simulink model "npc_controller"  (R2022a)
settings: Solver=FixedStepDiscrete  StartTime=0.0  StopTime=20  RelTol=1e-3  EnableMultiTasking=on
values from neighbouring files (symbols this model uses):
  Tsw = 1.5E-5    [param.sldd]
undefined symbols (not defined in the file or in its folder): CAN_O_INT, CANA_BASE, Down, GPTRIP1SEL, GPTRIP2SEL, GPTRIP3SEL, TZ1, TZ2, TZ3, Up
libraries: simulink x153, hdlsllib x90, c2802xlib x34, c2837xDlib x18, c280xlib x12, canmsglib x9, c2838xlib x8, idelinklib_common x3, c2806xlib x2, slpidlib x2, c28004xlib x2, c281xlib x2
(part 32 of 45)

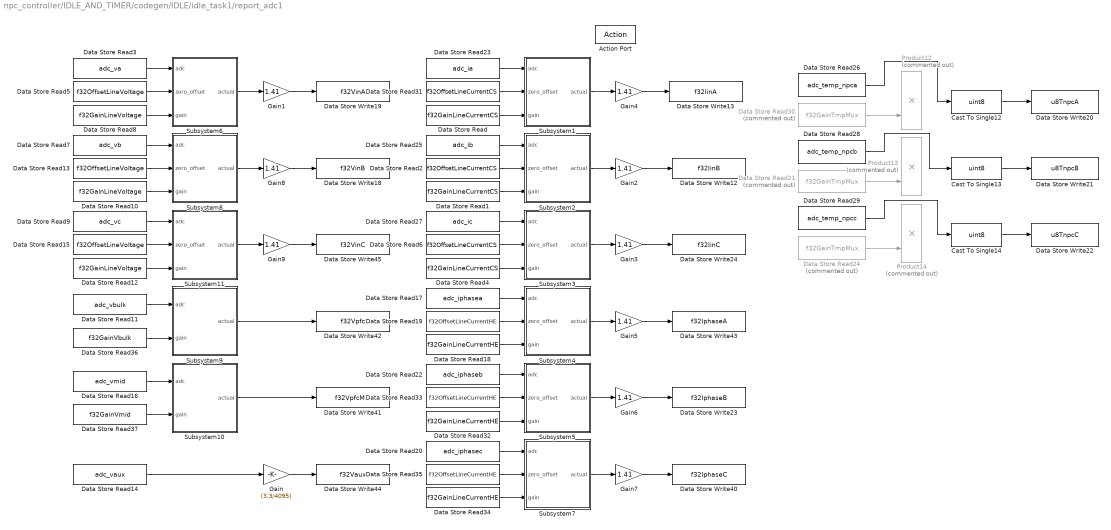
== system npc_controller/IDLE_AND_TIMER/codegen/IDLE/idle_task1/report_adc1 ==
  Action Port : ActionPort
  Cast To Single12 : DataTypeConversion  OutDataTypeStr=uint8  SaturateOnIntegerOverflow=off  RndMeth=Floor
  Cast To Single13 : DataTypeConversion  OutDataTypeStr=uint8  SaturateOnIntegerOverflow=off  RndMeth=Floor
  Cast To Single14 : DataTypeConversion  OutDataTypeStr=uint8  SaturateOnIntegerOverflow=off  RndMeth=Floor
  Data Store Read : DataStoreRead  DataStoreName=f32GainLineCurrentCS  IndexOptions=Index vector (dialog)  Indices=1  OutputSizes=1
  Data Store Read1 : DataStoreRead  DataStoreName=f32GainLineCurrentCS  IndexOptions=Index vector (dialog)  Indices=1  OutputSizes=1
  Data Store Read10 : DataStoreRead  DataStoreName=f32GainLineVoltage  IndexOptions=Index vector (dialog)  Indices=1  OutputSizes=1
  Data Store Read11 : DataStoreRead  DataStoreName=adc_vbulk  IndexOptions=Index vector (dialog)  Indices=1  OutputSizes=1
  Data Store Read12 : DataStoreRead  DataStoreName=f32GainLineVoltage  IndexOptions=Index vector (dialog)  Indices=1  OutputSizes=1
  Data Store Read13 : DataStoreRead  DataStoreName=f32OffsetLineVoltage  IndexOptions=Index vector (dialog)  Indices=1  OutputSizes=1
  Data Store Read14 : DataStoreRead  DataStoreName=adc_vaux  IndexOptions=Index vector (dialog)  Indices=1  OutputSizes=1
  Data Store Read15 : DataStoreRead  DataStoreName=f32OffsetLineVoltage  IndexOptions=Index vector (dialog)  Indices=1  OutputSizes=1
  Data Store Read16 : DataStoreRead  DataStoreName=adc_vmid  IndexOptions=Index vector (dialog)  Indices=1  OutputSizes=1
  Data Store Read17 : DataStoreRead  DataStoreName=adc_iphasea  IndexOptions=Index vector (dialog)  Indices=1  OutputSizes=1
  Data Store Read18 : DataStoreRead  DataStoreName=f32GainLineCurrentHE  IndexOptions=Index vector (dialog)  Indices=1  OutputSizes=1
  Data Store Read19 : DataStoreRead  DataStoreName=f32OffsetLineCurrentHE  IndexOptions=Index vector (dialog)  Indices=1  OutputSizes=1
  Data Store Read2 : DataStoreRead  DataStoreName=f32OffsetLineCurrentCS  IndexOptions=Index vector (dialog)  Indices=1  OutputSizes=1
  Data Store Read20 : DataStoreRead  DataStoreName=adc_iphasec  IndexOptions=Index vector (dialog)  Indices=1  OutputSizes=1
  Data Store Read21 : DataStoreRead  Commented=on  DataStoreName=f32GainTmpMux  IndexOptions=Index vector (dialog)  Indices=1  OutputSizes=1
  Data Store Read22 : DataStoreRead  DataStoreName=adc_iphaseb  IndexOptions=Index vector (dialog)  Indices=1  OutputSizes=1
  Data Store Read23 : DataStoreRead  DataStoreName=adc_ia  IndexOptions=Index vector (dialog)  Indices=1  OutputSizes=1
  Data Store Read24 : DataStoreRead  Commented=on  DataStoreName=f32GainTmpMux  IndexOptions=Index vector (dialog)  Indices=1  OutputSizes=1
  Data Store Read25 : DataStoreRead  DataStoreName=adc_ib  IndexOptions=Index vector (dialog)  Indices=1  OutputSizes=1
  Data Store Read26 : DataStoreRead  DataStoreName=adc_temp_npca  IndexOptions=Index vector (dialog)  Indices=1  OutputSizes=1
  Data Store Read27 : DataStoreRead  DataStoreName=adc_ic  IndexOptions=Index vector (dialog)  Indices=1  OutputSizes=1
  Data Store Read28 : DataStoreRead  DataStoreName=adc_temp_npcb  IndexOptions=Index vector (dialog)  Indices=1  OutputSizes=1
  Data Store Read29 : DataStoreRead  DataStoreName=adc_temp_npcc  IndexOptions=Index vector (dialog)  Indices=1  OutputSizes=1
  Data Store Read3 : DataStoreRead  DataStoreName=adc_va  IndexOptions=Index vector (dialog)  Indices=1  OutputSizes=1
  Data Store Read30 : DataStoreRead  Commented=on  DataStoreName=f32GainTmpMux  IndexOptions=Index vector (dialog)  Indices=1  OutputSizes=1
  Data Store Read31 : DataStoreRead  DataStoreName=f32OffsetLineCurrentCS  IndexOptions=Index vector (dialog)  Indices=1  OutputSizes=1
  Data Store Read32 : DataStoreRead  DataStoreName=f32GainLineCurrentHE  IndexOptions=Index vector (dialog)  Indices=1  OutputSizes=1
  Data Store Read33 : DataStoreRead  DataStoreName=f32OffsetLineCurrentHE  IndexOptions=Index vector (dialog)  Indices=1  OutputSizes=1
  Data Store Read34 : DataStoreRead  DataStoreName=f32GainLineCurrentHE  IndexOptions=Index vector (dialog)  Indices=1  OutputSizes=1
  Data Store Read35 : DataStoreRead  DataStoreName=f32OffsetLineCurrentHE  IndexOptions=Index vector (dialog)  Indices=1  OutputSizes=1
  Data Store Read36 : DataStoreRead  DataStoreName=f32GainVbulk  IndexOptions=Index vector (dialog)  Indices=1  OutputSizes=1
  Data Store Read37 : DataStoreRead  DataStoreName=f32GainVmid  IndexOptions=Index vector (dialog)  Indices=1  OutputSizes=1
  Data Store Read4 : DataStoreRead  DataStoreName=f32GainLineCurrentCS  IndexOptions=Index vector (dialog)  Indices=1  OutputSizes=1
  Data Store Read5 : DataStoreRead  DataStoreName=f32OffsetLineVoltage  IndexOptions=Index vector (dialog)  Indices=1  OutputSizes=1
  Data Store Read6 : DataStoreRead  DataStoreName=f32OffsetLineCurrentCS  IndexOptions=Index vector (dialog)  Indices=1  OutputSizes=1
  Data Store Read7 : DataStoreRead  DataStoreName=adc_vb  IndexOptions=Index vector (dialog)  Indices=1  OutputSizes=1
  Data Store Read8 : DataStoreRead  DataStoreName=f32GainLineVoltage  IndexOptions=Index vector (dialog)  Indices=1  OutputSizes=1
  Data Store Read9 : DataStoreRead  DataStoreName=adc_vc  IndexOptions=Index vector (dialog)  Indices=1  OutputSizes=1
  Data Store Write12 : DataStoreWrite  DataStoreName=f32IinB  IndexOptions=Index vector (dialog)  Indices=1  OutputSizes=1
  Data Store Write13 : DataStoreWrite  DataStoreName=f32IinA  IndexOptions=Index vector (dialog)  Indices=1  OutputSizes=1
  Data Store Write18 : DataStoreWrite  DataStoreName=f32VinB  IndexOptions=Index vector (dialog)  Indices=1  OutputSizes=1
  Data Store Write19 : DataStoreWrite  DataStoreName=f32VinA  IndexOptions=Index vector (dialog)  Indices=1  OutputSizes=1
  Data Store Write20 : DataStoreWrite  DataStoreName=u8TnpcA  IndexOptions=Index vector (dialog)  Indices=1  OutputSizes=1
  Data Store Write21 : DataStoreWrite  DataStoreName=u8TnpcB  IndexOptions=Index vector (dialog)  Indices=1  OutputSizes=1
  Data Store Write22 : DataStoreWrite  DataStoreName=u8TnpcC  IndexOptions=Index vector (dialog)  Indices=1  OutputSizes=1
  Data Store Write23 : DataStoreWrite  DataStoreName=f32IphaseB  IndexOptions=Index vector (dialog)  Indices=1  OutputSizes=1
  Data Store Write24 : DataStoreWrite  DataStoreName=f32IinC  IndexOptions=Index vector (dialog)  Indices=1  OutputSizes=1
  Data Store Write40 : DataStoreWrite  DataStoreName=f32IphaseC  IndexOptions=Index vector (dialog)  Indices=1  OutputSizes=1
  Data Store Write41 : DataStoreWrite  DataStoreName=f32VpfcMid  IndexOptions=Index vector (dialog)  Indices=1  OutputSizes=1
  Data Store Write42 : DataStoreWrite  DataStoreName=f32Vpfc  IndexOptions=Index vector (dialog)  Indices=1  OutputSizes=1
  Data Store Write43 : DataStoreWrite  DataStoreName=f32IphaseA  IndexOptions=Index vector (dialog)  Indices=1  OutputSizes=1
  Data Store Write44 : DataStoreWrite  DataStoreName=f32Vaux  IndexOptions=Index vector (dialog)  Indices=1  OutputSizes=1
  Data Store Write45 : DataStoreWrite  DataStoreName=f32VinC  IndexOptions=Index vector (dialog)  Indices=1  OutputSizes=1
  Gain : Gain  Gain=(3.3/4095)  ParamDataTypeStr=single  OutDataTypeStr=single
  Gain{1..9} (9 alike) : Gain  Gain=1.41  ParamDataTypeStr=single  OutDataTypeStr=single
  Product12 : Product  Commented=on  OutDataTypeStr=single
  Product13 : Product  Commented=on  OutDataTypeStr=single
  Product14 : Product  Commented=on  OutDataTypeStr=single
  Subsystem1 : Subsystem
  Subsystem10 : Subsystem
  Subsystem11 : Subsystem
  Subsystem2 : Subsystem
  Subsystem3 : Subsystem
  Subsystem4 : Subsystem
  Subsystem5 : Subsystem
  Subsystem6 : Subsystem
  Subsystem7 : Subsystem
  Subsystem8 : Subsystem
  Subsystem9 : Subsystem
  wires:
  Data Store Read3/1 -> Subsystem6/1(adc)
  Subsystem8/1(actual) -> Gain8/1
  Subsystem11/1(actual) -> Gain9/1
  Subsystem5/1(actual) -> Gain6/1
  Subsystem7/1(actual) -> Gain7/1
  Subsystem4/1(actual) -> Gain5/1
  Subsystem3/1(actual) -> Gain3/1
  Subsystem2/1(actual) -> Gain2/1
  Gain7/1 -> Data Store Write40/1
  Gain6/1 -> Data Store Write23/1
  Gain5/1 -> Data Store Write43/1
  Gain3/1 -> Data Store Write24/1
  Subsystem9/1(actual) -> Data Store Write42/1
  Data Store Read23/1 -> Subsystem1/1(adc)
  Gain1/1 -> Data Store Write19/1
  Subsystem6/1(actual) -> Gain1/1
  Gain2/1 -> Data Store Write12/1
  Gain4/1 -> Data Store Write13/1
  Subsystem10/1(actual) -> Data Store Write41/1
  Gain9/1 -> Data Store Write45/1
  Gain8/1 -> Data Store Write18/1
  Data Store Read29/1 -> Cast To Single14/1
  Data Store Read28/1 -> Cast To Single13/1
  Data Store Read26/1 -> Cast To Single12/1
  Data Store Read13/1 -> Subsystem8/2(zero_offset)
  Data Store Read10/1 -> Subsystem8/3(gain)
  Data Store Read31/1 -> Subsystem1/2(zero_offset)
  Data Store Read/1 -> Subsystem1/3(gain)
  Data Store Read8/1 -> Subsystem6/3(gain)
  Data Store Read5/1 -> Subsystem6/2(zero_offset)
  Gain/1 -> Data Store Write44/1
  Data Store Read37/1 -> Subsystem10/2(gain)
  Data Store Read36/1 -> Subsystem9/2(gain)
  Data Store Read12/1 -> Subsystem11/3(gain)
  Data Store Read15/1 -> Subsystem11/2(zero_offset)
  Data Store Read16/1 -> Subsystem10/1(adc)
  Data Store Read11/1 -> Subsystem9/1(adc)
  Data Store Read9/1 -> Subsystem11/1(adc)
  Data Store Read7/1 -> Subsystem8/1(adc)
  Data Store Read34/1 -> Subsystem7/3(gain)
  Data Store Read35/1 -> Subsystem7/2(zero_offset)
  Data Store Read33/1 -> Subsystem5/2(zero_offset)
  Data Store Read32/1 -> Subsystem5/3(gain)
  Data Store Read18/1 -> Subsystem4/3(gain)
  Data Store Read19/1 -> Subsystem4/2(zero_offset)
  Data Store Read4/1 -> Subsystem3/3(gain)
  Data Store Read6/1 -> Subsystem3/2(zero_offset)
  Data Store Read1/1 -> Subsystem2/3(gain)
  Data Store Read2/1 -> Subsystem2/2(zero_offset)
  Data Store Read20/1 -> Subsystem7/1(adc)
  Data Store Read22/1 -> Subsystem5/1(adc)
  Data Store Read17/1 -> Subsystem4/1(adc)
  Data Store Read27/1 -> Subsystem3/1(adc)
  Data Store Read25/1 -> Subsystem2/1(adc)
  Subsystem1/1(actual) -> Gain4/1
  Data Store Read24/1 -> Product14/2
  Data Store Read21/1 -> Product13/2
  Data Store Read30/1 -> Product12/2
  Cast To Single12/1 -> Data Store Write20/1
  Cast To Single14/1 -> Data Store Write22/1
  Cast To Single13/1 -> Data Store Write21/1
  Data Store Read14/1 -> Gain/1

== system npc_controller/IDLE_AND_TIMER/codegen/IDLE/idle_task1/set_tmp_mux ==
  Action Port : ActionPort  ActionPortLabel=case [ 3 ]:
  Function-Call Generator : simulink/Ports & Subsystems/Function-Call Generator  sample_time=-1  numberOfIterations=1  DisallowWideOutput=off
  Function-Call Split : FunctionCallSplit  NumOutputPorts=2
  Function-Call Split1 : FunctionCallSplit  NumOutputPorts=2
  incr_cnt_tmp_mux : Subsystem  TreatAsAtomicUnit=on
      settings: RTWSystemCode=Inline
  parse_cnt_tmp_mux : Subsystem  TreatAsAtomicUnit=on
      settings: RTWSystemCode=Inline
  set_tmp_mux : Subsystem
  wires:
  Function-Call Generator/1 -> Function-Call Split/1
  Function-Call Split/1 -> parse_cnt_tmp_mux/Trigger
  Function-Call Split1/2 -> incr_cnt_tmp_mux/Trigger
  Function-Call Split1/1 -> set_tmp_mux/Trigger
  Function-Call Split/2 -> Function-Call Split1/1

== system npc_controller/IDLE_AND_TIMER/codegen/IDLE/idle_task1/watchdog ==
  note: Note add MLE
  Action Port : ActionPort  ActionPortLabel=case [ 0 ]:
  Watchdog : c281xlib/Watchdog  resetsrc=Specify via dialog  sample=-1
      settings: SourceProductBaseCode=TIC2000

== system npc_controller/IDLE_AND_TIMER/codegen/INITIALIZATION/clb/System Initialize1 ==

== system npc_controller/IDLE_AND_TIMER/codegen/INITIALIZATION/clb/System Initialize2 ==

== system npc_controller/IDLE_AND_TIMER/codegen/INITIALIZATION/clb/System Initialize8 ==

== system npc_controller/IDLE_AND_TIMER/codegen/INITIALIZATION/epwm/System Initialize3 ==

== system npc_controller/IDLE_AND_TIMER/codegen/INITIALIZATION/epwm1/System Initialize1 ==

== system npc_controller/IDLE_AND_TIMER/codegen/INITIALIZATION/epwm1/System Initialize3 ==

== system npc_controller/IDLE_AND_TIMER/codegen/INITIALIZATION/outputxbar/System Initialize1 ==

== system npc_controller/IDLE_AND_TIMER/codegen/INITIALIZATION/outputxbar/System Initialize2 ==

== system npc_controller/IDLE_AND_TIMER/codegen/INITIALIZATION/outputxbar/System Initialize3 ==

== system npc_controller/IDLE_AND_TIMER/codegen/INITIALIZATION/outputxbar/System Initialize4 ==

== system npc_controller/IDLE_AND_TIMER/codegen/INITIALIZATION/outputxbar/System Initialize5 ==

== system npc_controller/IDLE_AND_TIMER/codegen/INITIALIZATION/outputxbar/System Initialize6 ==

== system npc_controller/IDLE_AND_TIMER/codegen/INITIALIZATION/outputxbar/System Initialize7 ==

== system npc_controller/IDLE_AND_TIMER/codegen/TIMER_100MS/incr_cnt/inc ==
  Action Port : ActionPort  ActionPortLabel=else
  Add : Sum
  Constant : Constant  OutDataTypeStr=uint16
  Data Store Read : DataStoreRead  DataStoreName=cnt_poll_can_msg  IndexOptions=Index vector (dialog)  Indices=1  OutputSizes=1
  Data Store Write : DataStoreWrite  DataStoreName=cnt_poll_can_msg  IndexOptions=Index vector (dialog)  Indices=1  OutputSizes=1
  wires:
  Add/1 -> Data Store Write/1
  Data Store Read/1 -> Add/1
  Constant/1 -> Add/2

== system npc_controller/IDLE_AND_TIMER/codegen/TIMER_100MS/incr_cnt/reset ==
  Action Port : ActionPort  ActionPortLabel=if(u1 > 10)
  Constant : Constant  Value=0  OutDataTypeStr=uint16
  Data Store Write : DataStoreWrite  DataStoreName=cnt_poll_can_msg  IndexOptions=Index vector (dialog)  Indices=1  OutputSizes=1
  wires:
  Constant/1 -> Data Store Write/1

== system npc_controller/IDLE_AND_TIMER/codegen/TIMER_1MS/codegen/periodic_timer1 ==
  note: Note:
      |  - Worst error of tfv is timer interval (1ms) + twice the execution of supervisory loop
      |  - Effective max count is 65.536 = 2e16*1e-3
  Add : Sum  Commented=on
  Add1 : Sum
  Constant : Constant  Commented=on  OutDataTypeStr=uint16
  Constant1 : Constant  OutDataTypeStr=uint16
  Data Store Read : DataStoreRead  Commented=on  DataStoreName=cnt_1ms  IndexOptions=Index vector (dialog)  Indices=1  OutputSizes=1
  Data Store Read1 : DataStoreRead  DataStoreName=cnt_1ms  IndexOptions=Index vector (dialog)  Indices=1  OutputSizes=1
  Data Store Write : DataStoreWrite  Commented=on  DataStoreName=cnt_1ms  IndexOptions=Index vector (dialog)  Indices=1  OutputSizes=1
  Data Store Write1 : DataStoreWrite  DataStoreName=cnt_1ms  IndexOptions=Index vector (dialog)  Indices=1  OutputSizes=1
  Rate Transition2 : RateTransition
  Rate Transition3 : RateTransition
  wires:
  Constant/1 -> Add/2
  Add/1 -> Data Store Write/1
  Data Store Read/1 -> Add/1
  Rate Transition3/1 -> Add1/1
  Rate Transition2/1 -> Data Store Write1/1
  Data Store Read1/1 -> Rate Transition3/1
  Add1/1 -> Rate Transition2/1
  Constant1/1 -> Add1/2

== system npc_controller/CONTROL/CONTROL/false/CLA_CONTROL/CONTROL/IIR Filter1 ==
  note: prev 0.98
  x[n] : Inport
  1 - Lambda : Gain  Gain=1-0.9996  ParamDataTypeStr=single  OutDataTypeStr=single
  Delay : Delay  DelayLength=1  StateName=vmid_delay2  StateMustResolveToSignalObject=on
  Delay1 : Delay  DelayLength=1  StateName=vmid_delay1  StateMustResolveToSignalObject=on
  Lambda : Gain  Gain=0.9996  ParamDataTypeStr=single  OutDataTypeStr=single
  Sum : Sum  Inputs=|++  AccumDataTypeStr=single  OutDataTypeStr=single
  y[n] : Outport
  wires:
  Delay/1 -> Lambda/1
  Lambda/1 -> Sum/2
  Sum/1 -> y[n]/1, Delay/1
  1 - Lambda/1 -> Sum/1
  x[n]/1 -> Delay1/1
  Delay1/1 -> 1 - Lambda/1

== system npc_controller/CONTROL/CONTROL/false/CLA_CONTROL/CONTROL/IIR Filter3 ==
  note: prev 0.98
  x[n] : Inport
  1 - Lambda : Gain  Gain=1-0.9996  ParamDataTypeStr=single  OutDataTypeStr=single
  Delay : Delay  DelayLength=1  StateName=vbulk_delay2  StateMustResolveToSignalObject=on
  Delay1 : Delay  DelayLength=1  StateName=vbulk_delay1  StateMustResolveToSignalObject=on
  Lambda : Gain  Gain=0.9996  ParamDataTypeStr=single  OutDataTypeStr=single
  Sum : Sum  Inputs=|++  AccumDataTypeStr=single  OutDataTypeStr=single
  y[n] : Outport
  wires:
  Delay/1 -> Lambda/1
  Lambda/1 -> Sum/2
  Sum/1 -> y[n]/1, Delay/1
  1 - Lambda/1 -> Sum/1
  x[n]/1 -> Delay1/1
  Delay1/1 -> 1 - Lambda/1

== system npc_controller/CONTROL/CONTROL/false/CLA_CONTROL/CONTROL/If Action Subsystem ==
  In1 : Inport
  Action Port : ActionPort  ActionPortLabel=if(u1 == 1)
  Out1 : Outport
  wires:
  In1/1 -> Out1/1

== system npc_controller/CONTROL/CONTROL/false/CLA_CONTROL/CONTROL/If Action Subsystem1 ==
  In1 : Inport
  Action Port : ActionPort  ActionPortLabel=else
  Out1 : Outport
  wires:
  In1/1 -> Out1/1

== system npc_controller/CONTROL/CONTROL/false/CLA_CONTROL/CONTROL/Subsystem1 ==
  note: Note:
      | pol_pha
      | 0 - pos
      | 1 - neg
  iLref : Inport
  vbal_coef : Inport  Port=2
  pol : Inport  Port=3
  AND4 : Logic  Operator=NAND  IconShape=distinctive  AllPortsSameDT=off  OutDataTypeStr=boolean
  AND5 : Logic  IconShape=distinctive  AllPortsSameDT=off  OutDataTypeStr=boolean
  Add : Sum  AccumDataTypeStr=single  OutDataTypeStr=single
  Constant4 : Constant  Value=2  OutDataTypeStr=single  SampleTime=-1
  From3 : From  Commented=on  GotoTag=iLref
  From4 : From  Commented=on  GotoTag=iLref_pos
  From5 : From  Commented=on  GotoTag=iLref_neg
  From52 : From  Commented=on  GotoTag=vbal_coef_top
  From53 : From  Commented=on  GotoTag=vbal_coef_bot
  Mux : Mux  Commented=on  Inputs=3
  Mux1 : Mux  Commented=on  Inputs=2
  Product{4..5,10..11} (4 alike) : Product  OutDataTypeStr=single
  Scope3 : Scope  Commented=on  NumInputPorts=2
  delVdc5 : Sum  Inputs=|+-  AccumDataTypeStr=single  OutDataTypeStr=single
  iLref_vbal : Outport
  wires:
  Mux/1 -> Scope3/2
  Mux1/1 -> Scope3/1
  From52/1 -> Mux1/1
  From53/1 -> Mux1/2
  From5/1 -> Mux/3
  From4/1 -> Mux/2
  From3/1 -> Mux/1
  pol/1 -> [pol]
  Add/1 -> iLref_vbal/1
  iLref/1 -> [iLref]
  vbal_coef/1 -> [vbal_coef_top]
  [vbal_coef_top] -> delVdc5/2
  Constant4/1 -> delVdc5/1
  delVdc5/1 -> [vbal_coef_bot]
  [iLref] -> AND5/1, Product11/1
  Product5/1 -> Add/2
  [iLref_pos] -> Product4/1
  [vbal_coef_top] -> Product4/2
  [iLref_neg] -> Product5/1
  AND4/1 -> Product10/2
  Product4/1 -> Add/1
  Product10/1 -> [iLref_pos]
  [pol] -> AND4/2
  [vbal_coef_bot] -> Product5/2
  [iLref] -> AND4/1, Product10/1
  AND5/1 -> Product11/2
  [pol] -> AND5/2
  Product11/1 -> [iLref_neg]

== system npc_controller/CONTROL/CONTROL/false/CLA_CONTROL/CONTROL/Subsystem2 ==
  note: Note:
      | pol_pha
      | 0 - pos
      | 1 - neg
  iLref : Inport
  vbal_coef : Inport  Port=2
  pol : Inport  Port=3
  AND4 : Logic  Operator=NAND  IconShape=distinctive  AllPortsSameDT=off  OutDataTypeStr=boolean
  AND5 : Logic  IconShape=distinctive  AllPortsSameDT=off  OutDataTypeStr=boolean
  Add : Sum  AccumDataTypeStr=single  OutDataTypeStr=single
  Constant4 : Constant  Value=2  OutDataTypeStr=single  SampleTime=-1
  From3 : From  Commented=on  GotoTag=iLref
  From4 : From  Commented=on  GotoTag=iLref_pos
  From5 : From  Commented=on  GotoTag=iLref_neg
  From52 : From  Commented=on  GotoTag=vbal_coef_top
  From53 : From  Commented=on  GotoTag=vbal_coef_bot
  Mux : Mux  Commented=on  Inputs=3
  Mux1 : Mux  Commented=on  Inputs=2
  Product{4..5,10..11} (4 alike) : Product  OutDataTypeStr=single
  Scope3 : Scope  Commented=on  NumInputPorts=2
  delVdc5 : Sum  Inputs=|+-  AccumDataTypeStr=single  OutDataTypeStr=single
  iLref_vbal : Outport
  wires:
  Product11/1 -> [iLref_neg]
  [pol] -> AND5/2
  AND5/1 -> Product11/2
  [iLref] -> Product10/1, AND4/1
  [vbal_coef_bot] -> Product5/2
  [pol] -> AND4/2
  Product10/1 -> [iLref_pos]
  Product4/1 -> Add/1
  AND4/1 -> Product10/2
  [iLref_neg] -> Product5/1
  [vbal_coef_top] -> Product4/2
  [iLref_pos] -> Product4/1
  Product5/1 -> Add/2
  [iLref] -> Product11/1, AND5/1
  delVdc5/1 -> [vbal_coef_bot]
  Constant4/1 -> delVdc5/1
  [vbal_coef_top] -> delVdc5/2
  vbal_coef/1 -> [vbal_coef_top]
  iLref/1 -> [iLref]
  Add/1 -> iLref_vbal/1
  pol/1 -> [pol]
  From3/1 -> Mux/1
  From4/1 -> Mux/2
  From5/1 -> Mux/3
  From53/1 -> Mux1/2
  From52/1 -> Mux1/1
  Mux1/1 -> Scope3/1
  Mux/1 -> Scope3/2

== system npc_controller/CONTROL/CONTROL/false/CLA_CONTROL/CONTROL/Subsystem5 ==
  vxn : Inport  OutDataTypeStr=single
  vbulk : Inport  Port=2  OutDataTypeStr=single
  iLxref : Inport  Port=3  OutDataTypeStr=single
  Constant4 : Constant  OutDataTypeStr=single  SampleTime=-1
  Delay : Delay  DelayLength=1  StateName=dcmccm_delay  StateMustResolveToSignalObject=on
  Divide6 : Product  Inputs=*/  OutDataTypeStr=single
  Divide7 : Product  Inputs=***/  OutDataTypeStr=single
  Gain10 : Gain  Gain=0.5  ParamDataTypeStr=single  OutDataTypeStr=single
  Gain11 : Gain  Gain=1538  ParamDataTypeStr=single  OutDataTypeStr=single
  Gain9 : Gain  Gain=0.0036102/0.001798  ParamDataTypeStr=single  OutDataTypeStr=single
  KL : Constant  Value=2.6305  OutDataTypeStr=single  SampleTime=-1
  Min : MinMax  Inputs=2  OutDataTypeStr=single
  Saturation2 : Saturate  UpperLimit=1  LowerLimit=0  OutDataTypeStr=single
  Saturation3 : Saturate  UpperLimit=1  LowerLimit=0  OutDataTypeStr=single
  Sqrt : Sqrt  OutputSignalType=real  OutDataTypeStr=single  IntermediateResultsDataTypeStr=single
  Sum7 : Sum  Inputs=|+-  AccumDataTypeStr=single  OutDataTypeStr=single
  D_FF : Outport  OutDataTypeStr=single
  wires:
  Gain10/1 -> Divide6/2
  Saturation2/1 -> Delay/1, Min/1  "D_CCM"
  vxn/1 -> Divide7/4, Gain9/1
  Gain9/1 -> Divide6/1
  Sqrt/1 -> Saturation3/1
  Sum7/1 -> Saturation2/1
  Gain11/1 -> D_FF/1  "D_FF"
  Divide7/1 -> Sqrt/1
  Saturation3/1 -> Min/2  "D_DCM"
  Divide6/1 -> Sum7/2
  Constant4/1 -> Sum7/1
  iLxref/1 -> Divide7/3
  Delay/1 -> Divide7/1
  Min/1 -> Gain11/1
  KL/1 -> Divide7/2
  vbulk/1 -> Gain10/1

== system npc_controller/CONTROL/CONTROL/false/CLA_CONTROL/CONTROL/midpoint voltage balancing ==
  note: Note:
      | pol_pha
      | 0 - pos
      | 1 - neg
  iLref : Inport
  vbal_coef : Inport  Port=2
  pol : Inport  Port=3
  AND4 : Logic  Operator=NAND  IconShape=distinctive  AllPortsSameDT=off  OutDataTypeStr=boolean
  AND5 : Logic  IconShape=distinctive  AllPortsSameDT=off  OutDataTypeStr=boolean
  Add : Sum  AccumDataTypeStr=single  OutDataTypeStr=single
  Constant4 : Constant  Value=2  OutDataTypeStr=single  SampleTime=-1
  From3 : From  Commented=on  GotoTag=iLref
  From4 : From  Commented=on  GotoTag=iLref_pos
  From5 : From  Commented=on  GotoTag=iLref_neg
  From52 : From  Commented=on  GotoTag=vbal_coef_top
  From53 : From  Commented=on  GotoTag=vbal_coef_bot
  Mux : Mux  Commented=on  Inputs=3
  Mux1 : Mux  Commented=on  Inputs=2
  Product{4..5,10..11} (4 alike) : Product  OutDataTypeStr=single
  Scope3 : Scope  Commented=on  NumInputPorts=2
  delVdc5 : Sum  Inputs=|+-  AccumDataTypeStr=single  OutDataTypeStr=single
  iLref_vbal : Outport
  wires:
  Product11/1 -> [iLref_neg]
  [pol] -> AND5/2
  AND5/1 -> Product11/2
  [iLref] -> Product10/1, AND4/1
  [vbal_coef_bot] -> Product5/2
  [pol] -> AND4/2
  Product10/1 -> [iLref_pos]
  Product4/1 -> Add/1
  AND4/1 -> Product10/2
  [iLref_neg] -> Product5/1
  [vbal_coef_top] -> Product4/2
  [iLref_pos] -> Product4/1
  Product5/1 -> Add/2
  [iLref] -> Product11/1, AND5/1
  delVdc5/1 -> [vbal_coef_bot]
  Constant4/1 -> delVdc5/1
  [vbal_coef_top] -> delVdc5/2
  vbal_coef/1 -> [vbal_coef_top]
  iLref/1 -> [iLref]
  Add/1 -> iLref_vbal/1
  pol/1 -> [pol]
  From3/1 -> Mux/1
  From4/1 -> Mux/2
  From5/1 -> Mux/3
  From53/1 -> Mux1/2
  From52/1 -> Mux1/1
  Mux1/1 -> Scope3/1
  Mux/1 -> Scope3/2

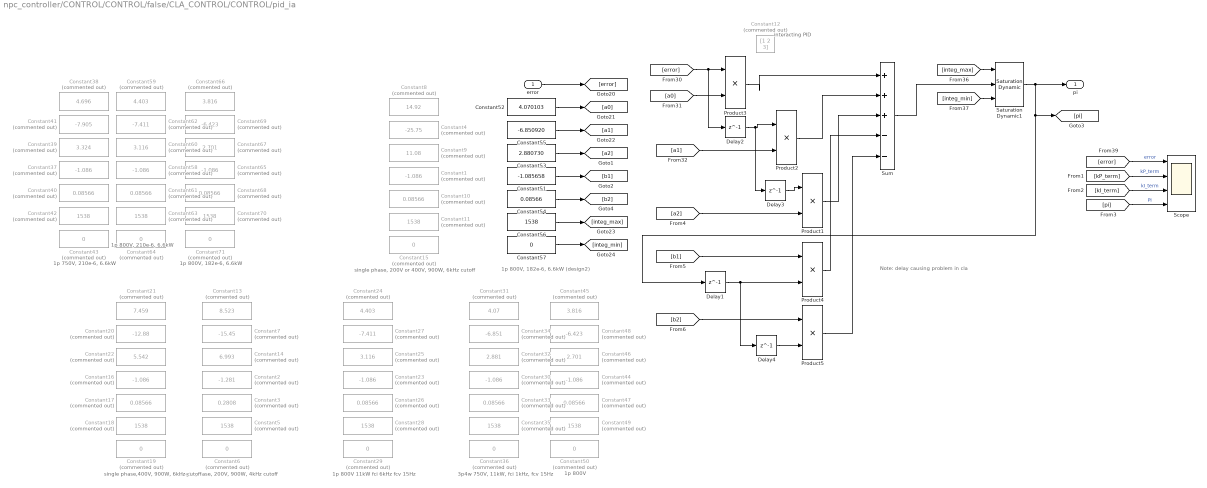
== system npc_controller/CONTROL/CONTROL/false/CLA_CONTROL/CONTROL/pid_ia ==
  note: single phase, 200V or 400V, 900W, 6kHz cutoff
  note: interacting PID
  note: Note: delay causing problem in cla
  note: single phase, 200V, 900W, 4kHz cutoff
  note: single phase,400V, 900W, 6kHz cutoff
  note: 1p 800V 11kW fci 6kHz fcv 15Hz
  note: 3p4w 750V, 11kW, fci 1kHz, fcv 15Hz
  note: 1p 750V, 210e-6, 6.6kW
  note: 1p 800V
  note: 1p 800V, 182e-6, 6.6kW (design2)
  note: 1p 800V, 210e-6, 6.6kW
  note: 1p 800V, 182e-6, 6.6kW
  error : Inport  OutDataTypeStr=single
  Constant{1,16,23,30,37,44,58,65} (8 alike) : Constant  Commented=on  Value=-1.086  OutDataTypeStr=single
  Constant{10,17,26,33,40,47,61,68} (8 alike) : Constant  Commented=on  Value=0.08566  OutDataTypeStr=single
  Constant{5,11,18,28,35,42,49,63,70} (9 alike) : Constant  Commented=on  Value=1538  OutDataTypeStr=single
  Constant12 : Constant  Commented=on  Value=[1 2 3]  OutDataTypeStr=single
  Constant13 : Constant  Commented=on  Value=8.523  VectorParams1D=off  OutDataTypeStr=single
  Constant14 : Constant  Commented=on  Value=6.993  OutDataTypeStr=single
  Constant{6,15,19,29,36,43,50,64,71} (9 alike) : Constant  Commented=on  Value=0  OutDataTypeStr=single
  Constant2 : Constant  Commented=on  Value=-1.281  OutDataTypeStr=single
  Constant20 : Constant  Commented=on  Value=-12.88  OutDataTypeStr=single
  Constant21 : Constant  Commented=on  Value=7.459  VectorParams1D=off  OutDataTypeStr=single
  Constant22 : Constant  Commented=on  Value=5.542  OutDataTypeStr=single
  Constant24 : Constant  Commented=on  Value=4.403  VectorParams1D=off  OutDataTypeStr=single
  Constant25 : Constant  Commented=on  Value=3.116  OutDataTypeStr=single
  Constant27 : Constant  Commented=on  Value=-7.411  OutDataTypeStr=single
  Constant3 : Constant  Commented=on  Value=0.2808  OutDataTypeStr=single
  Constant31 : Constant  Commented=on  Value=4.07  VectorParams1D=off  OutDataTypeStr=single
  Constant32 : Constant  Commented=on  Value=2.881  OutDataTypeStr=single
  Constant34 : Constant  Commented=on  Value=-6.851  OutDataTypeStr=single
  Constant38 : Constant  Commented=on  Value=4.696  VectorParams1D=off  OutDataTypeStr=single
  Constant39 : Constant  Commented=on  Value=3.324  OutDataTypeStr=single
  Constant4 : Constant  Commented=on  Value=-25.75  OutDataTypeStr=single
  Constant41 : Constant  Commented=on  Value=-7.905  OutDataTypeStr=single
  Constant45 : Constant  Commented=on  Value=3.816  VectorParams1D=off  OutDataTypeStr=single
  Constant46 : Constant  Commented=on  Value=2.701  OutDataTypeStr=single
  Constant48 : Constant  Commented=on  Value=-6.423  OutDataTypeStr=single
  Constant51 : Constant  Value=-1.085658  OutDataTypeStr=single
  Constant52 : Constant  Value=4.070103  VectorParams1D=off  OutDataTypeStr=single
  Constant53 : Constant  Value=2.880730  OutDataTypeStr=single
  Constant54 : Constant  Value=0.08566  OutDataTypeStr=single
  Constant55 : Constant  Value=-6.850920  OutDataTypeStr=single
  Constant56 : Constant  Value=1538  OutDataTypeStr=single
  Constant57 : Constant  Value=0  OutDataTypeStr=single
  Constant59 : Constant  Commented=on  Value=4.403  VectorParams1D=off  OutDataTypeStr=single
  Constant60 : Constant  Commented=on  Value=3.116  OutDataTypeStr=single
  Constant62 : Constant  Commented=on  Value=-7.411  OutDataTypeStr=single
  Constant66 : Constant  Commented=on  Value=3.816  VectorParams1D=off  OutDataTypeStr=single
  Constant67 : Constant  Commented=on  Value=2.701  OutDataTypeStr=single
  Constant69 : Constant  Commented=on  Value=-6.423  OutDataTypeStr=single
  Constant7 : Constant  Commented=on  Value=-15.45  OutDataTypeStr=single
  Constant8 : Constant  Commented=on  Value=14.92  VectorParams1D=off  OutDataTypeStr=single
  Constant9 : Constant  Commented=on  Value=11.08  OutDataTypeStr=single
  Delay1 : Delay  DelayLength=1  InitialCondition=0  StateName=ia_pid3  StateMustResolveToSignalObject=on
  Delay2 : Delay  DelayLength=1  InitialCondition=0  StateName=ia_pid1  StateMustResolveToSignalObject=on
  Delay3 : Delay  DelayLength=1  InitialCondition=0  StateName=ia_pid2  StateMustResolveToSignalObject=on
  Delay4 : Delay  DelayLength=1  InitialCondition=0  StateName=ia_pid4  StateMustResolveToSignalObject=on
  Product{1..5} (5 alike) : Product  OutDataTypeStr=single
  Saturation Dynamic1 : simulink/Discontinuities/Saturation Dynamic  OutMin=[]  OutMax=[]  OutDataTypeStr=single  OutputDataTypeScalingMode=single  OutDataType=fixdt(1, 16)  OutScaling=2^-10  DoSatur=off
  Scope : Scope  NumInputPorts=4
  Sum : Sum  Inputs=|+++--  AccumDataTypeStr=single  OutDataTypeStr=single
  pi : Outport
  wires:
  Constant54/1 -> [b2]
  Constant53/1 -> [a2]
  Constant51/1 -> [b1]
  [b2] -> Product5/1
  Product4/1 -> Sum/4
  Product5/1 -> Sum/5
  Delay4/1 -> Product5/2
  [b1] -> Product4/1
  Delay1/1 -> Delay4/1, Product4/2
  Product1/1 -> Sum/3
  Product2/1 -> Sum/2
  Product3/1 -> Sum/1
  [a2] -> Product1/2
  Delay3/1 -> Product1/1
  Saturation Dynamic1/1 -> [pi], Delay1/1, pi/1
  Delay2/1 -> Delay3/1, Product2/1
  [error] -> Product3/1, Delay2/1
  Constant52/1 -> [a0]
  [a1] -> Product2/2
  error/1 -> [error]
  Constant55/1 -> [a1]
  Constant57/1 -> [integ_min]
  Constant56/1 -> [integ_max]
  [integ_max] -> Saturation Dynamic1/1
  [integ_min] -> Saturation Dynamic1/3
  Sum/1 -> Saturation Dynamic1/2
  [a0] -> Product3/2
  [pi] -> Scope/4  "PI"
  [kI_term] -> Scope/3  "kI_term"
  [kP_term] -> Scope/2  "kP_term"
  [error] -> Scope/1  "error"

== system npc_controller/CONTROL/CONTROL/false/CLA_CONTROL/CONTROL/pid_ib ==
  note: Note: delay causing problem in cla
  note: interacting PID
  note: 1p 800V, 182e-6, 6.6kW
  note: single phase, 200V or 400V, 900W, 6kHz cutoff
  note: 1p 800V, 182e-6, 6.6kW (design2)
  error : Inport  OutDataTypeStr=single
  Constant1 : Constant  Commented=on  Value=-1.086  OutDataTypeStr=single
  Constant10 : Constant  Commented=on  Value=0.08566  OutDataTypeStr=single
  Constant11 : Constant  Commented=on  Value=1538  OutDataTypeStr=single
  Constant12 : Constant  Commented=on  Value=[1 2 3]  OutDataTypeStr=single
  Constant13 : Constant  Value=1538  OutDataTypeStr=single
  Constant14 : Constant  Value=0  OutDataTypeStr=single
  Constant15 : Constant  Commented=on  Value=0  OutDataTypeStr=single
  Constant2 : Constant  Value=-1.085658  OutDataTypeStr=single
  Constant3 : Constant  Value=4.070103  VectorParams1D=off  OutDataTypeStr=single
  Constant4 : Constant  Commented=on  Value=-25.75  OutDataTypeStr=single
  Constant5 : Constant  Value=2.880730  OutDataTypeStr=single
  Constant51 : Constant  Commented=on  Value=-1.086  OutDataTypeStr=single
  Constant52 : Constant  Commented=on  Value=3.816  VectorParams1D=off  OutDataTypeStr=single
  Constant53 : Constant  Commented=on  Value=2.701  OutDataTypeStr=single
  Constant54 : Constant  Commented=on  Value=0.08566  OutDataTypeStr=single
  Constant55 : Constant  Commented=on  Value=-6.423  OutDataTypeStr=single
  Constant56 : Constant  Commented=on  Value=1538  OutDataTypeStr=single
  Constant57 : Constant  Commented=on  Value=0  OutDataTypeStr=single
  Constant6 : Constant  Value=0.08566  OutDataTypeStr=single
  Constant7 : Constant  Value=-6.850920  OutDataTypeStr=single
  Constant8 : Constant  Commented=on  Value=14.92  VectorParams1D=off  OutDataTypeStr=single
  Constant9 : Constant  Commented=on  Value=11.08  OutDataTypeStr=single
  Delay1 : Delay  DelayLength=1  InitialCondition=0  StateName=ib_pid3  StateMustResolveToSignalObject=on
  Delay2 : Delay  DelayLength=1  InitialCondition=0  StateName=ib_pid1  StateMustResolveToSignalObject=on
  Delay3 : Delay  DelayLength=1  InitialCondition=0  StateName=ib_pid2  StateMustResolveToSignalObject=on
  Delay4 : Delay  DelayLength=1  InitialCondition=0  StateName=ib_pid4  StateMustResolveToSignalObject=on
  Product{1..5} (5 alike) : Product  OutDataTypeStr=single
  Saturation Dynamic1 : simulink/Discontinuities/Saturation Dynamic  OutMin=[]  OutMax=[]  OutDataTypeStr=single  OutputDataTypeScalingMode=single  OutDataType=fixdt(1, 16)  OutScaling=2^-10  DoSatur=off
  Scope : Scope  NumInputPorts=4
  Sum : Sum  Inputs=|+++--  AccumDataTypeStr=single  OutDataTypeStr=single
  pi : Outport
  wires:
  [error] -> Scope/1  "error"
  [kP_term] -> Scope/2  "kP_term"
  [kI_term] -> Scope/3  "kI_term"
  [pi] -> Scope/4  "PI"
  [a0] -> Product3/2
  Sum/1 -> Saturation Dynamic1/2
  [integ_min] -> Saturation Dynamic1/3
  [integ_max] -> Saturation Dynamic1/1
  error/1 -> [error]
  [a1] -> Product2/2
  [error] -> Delay2/1, Product3/1
  Delay2/1 -> Product2/1, Delay3/1
  Saturation Dynamic1/1 -> pi/1, Delay1/1, [pi]
  Delay3/1 -> Product1/1
  [a2] -> Product1/2
  Product3/1 -> Sum/1
  Product2/1 -> Sum/2
  Product1/1 -> Sum/3
  Delay1/1 -> Product4/2, Delay4/1
  [b1] -> Product4/1
  Delay4/1 -> Product5/2
  Product5/1 -> Sum/5
  Product4/1 -> Sum/4
  [b2] -> Product5/1
  Constant3/1 -> [a0]
  Constant7/1 -> [a1]
  Constant5/1 -> [a2]
  Constant2/1 -> [b1]
  Constant6/1 -> [b2]
  Constant13/1 -> [integ_max]
  Constant14/1 -> [integ_min]

== system npc_controller/CONTROL/CONTROL/false/CLA_CONTROL/CONTROL/pid_ic ==
  note: interacting PID
  note: Note: delay causing problem in cla
  note: 1p 800V, 182e-6, 6.6kW
  note: single phase, 200V or 400V, 900W, 6kHz cutoff
  note: 1p 800V, 182e-6, 6.6kW (design2)
  error : Inport  OutDataTypeStr=single
  Constant1 : Constant  Commented=on  Value=-1.086  OutDataTypeStr=single
  Constant10 : Constant  Commented=on  Value=0.08566  OutDataTypeStr=single
  Constant11 : Constant  Commented=on  Value=1538  OutDataTypeStr=single
  Constant12 : Constant  Commented=on  Value=[1 2 3]  OutDataTypeStr=single
  Constant13 : Constant  Value=1538  OutDataTypeStr=single
  Constant14 : Constant  Value=0  OutDataTypeStr=single
  Constant15 : Constant  Commented=on  Value=0  OutDataTypeStr=single
  Constant2 : Constant  Value=-1.085658  OutDataTypeStr=single
  Constant3 : Constant  Value=4.070103  VectorParams1D=off  OutDataTypeStr=single
  Constant4 : Constant  Commented=on  Value=-25.75  OutDataTypeStr=single
  Constant5 : Constant  Value=2.880730  OutDataTypeStr=single
  Constant51 : Constant  Commented=on  Value=-1.086  OutDataTypeStr=single
  Constant52 : Constant  Commented=on  Value=3.816  VectorParams1D=off  OutDataTypeStr=single
  Constant53 : Constant  Commented=on  Value=2.701  OutDataTypeStr=single
  Constant54 : Constant  Commented=on  Value=0.08566  OutDataTypeStr=single
  Constant55 : Constant  Commented=on  Value=-6.423  OutDataTypeStr=single
  Constant56 : Constant  Commented=on  Value=1538  OutDataTypeStr=single
  Constant57 : Constant  Commented=on  Value=0  OutDataTypeStr=single
  Constant6 : Constant  Value=0.08566  OutDataTypeStr=single
  Constant7 : Constant  Value=-6.850920  OutDataTypeStr=single
  Constant8 : Constant  Commented=on  Value=14.92  VectorParams1D=off  OutDataTypeStr=single
  Constant9 : Constant  Commented=on  Value=11.08  OutDataTypeStr=single
  Delay1 : Delay  DelayLength=1  InitialCondition=0  StateName=ic_pid3  StateMustResolveToSignalObject=on
  Delay2 : Delay  DelayLength=1  InitialCondition=0  StateName=ic_pid1  StateMustResolveToSignalObject=on
  Delay3 : Delay  DelayLength=1  InitialCondition=0  StateName=ic_pid2  StateMustResolveToSignalObject=on
  Delay4 : Delay  DelayLength=1  InitialCondition=0  StateName=ic_pid4  StateMustResolveToSignalObject=on
  Product{1..5} (5 alike) : Product  OutDataTypeStr=single
  Saturation Dynamic1 : simulink/Discontinuities/Saturation Dynamic  OutMin=[]  OutMax=[]  OutDataTypeStr=single  OutputDataTypeScalingMode=single  OutDataType=fixdt(1, 16)  OutScaling=2^-10  DoSatur=off
  Scope : Scope  NumInputPorts=4
  Sum : Sum  Inputs=|+++--  AccumDataTypeStr=single  OutDataTypeStr=single
  pi : Outport
  wires:
  Constant6/1 -> [b2]
  Constant5/1 -> [a2]
  Constant2/1 -> [b1]
  [b2] -> Product5/1
  Product4/1 -> Sum/4
  Product5/1 -> Sum/5
  Delay4/1 -> Product5/2
  [b1] -> Product4/1
  Delay1/1 -> Delay4/1, Product4/2
  Product1/1 -> Sum/3
  Product2/1 -> Sum/2
  Product3/1 -> Sum/1
  [a2] -> Product1/2
  Delay3/1 -> Product1/1
  Saturation Dynamic1/1 -> [pi], Delay1/1, pi/1
  Delay2/1 -> Delay3/1, Product2/1
  [error] -> Product3/1, Delay2/1
  Constant3/1 -> [a0]
  [a1] -> Product2/2
  error/1 -> [error]
  Constant7/1 -> [a1]
  Constant14/1 -> [integ_min]
  Constant13/1 -> [integ_max]
  [integ_max] -> Saturation Dynamic1/1
  [integ_min] -> Saturation Dynamic1/3
  Sum/1 -> Saturation Dynamic1/2
  [a0] -> Product3/2
  [pi] -> Scope/4  "PI"
  [kI_term] -> Scope/3  "kI_term"
  [kP_term] -> Scope/2  "kP_term"
  [error] -> Scope/1  "error"
